simulink model "winder"  (R2025a)
settings: Solver=ode15s  StartTime=0.0  StopTime=Time.sim_time  FixedStep=Time.step_size  MaxStep=1e-4  RelTol=1e-3
values from neighbouring files (symbols this model uses):
  theta_table = Cam.theta_full    [winder_init.m]
  z_table = Cam.z_full    [winder_init.m]
undefined symbols (not defined in the file or in its folder): Cam, Core, Dancer, DC, Speed, Spool, Stepp, Tension, Wire
libraries: slpidlib x1
settings Model: Creator=psyco  LastModifiedBy=psyco

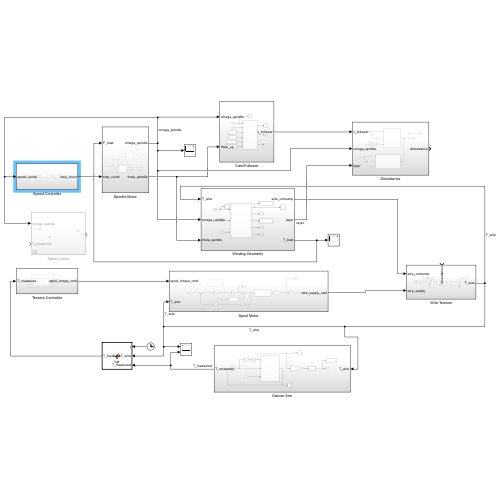
[thumbnail: Simulink's stored preview of the top-level diagram]
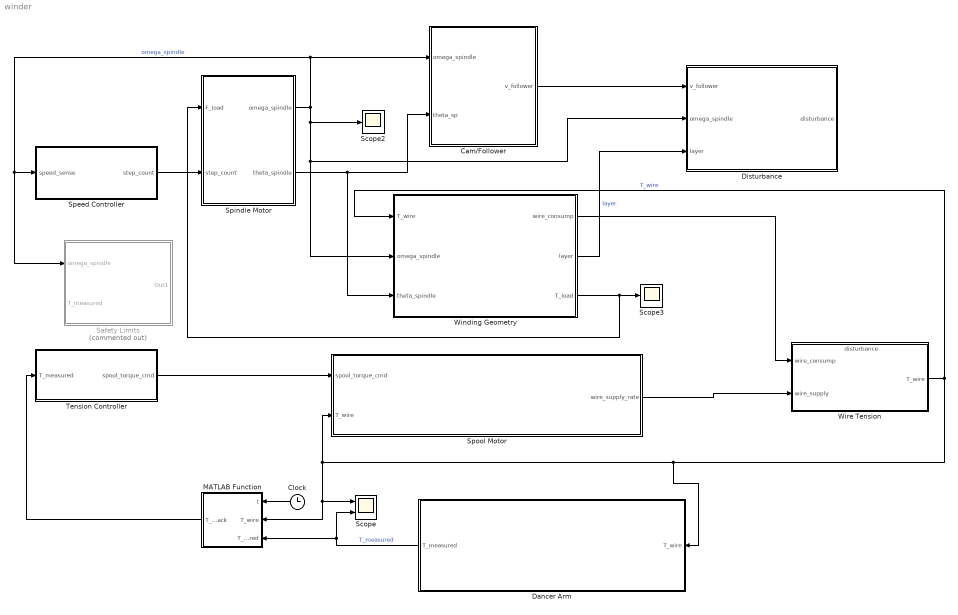
== system winder ==
  Cam/Follower : Subsystem
  Clock : Clock
  Dancer Arm : Subsystem
  Disturbance : Subsystem
  MATLAB Function : MATLAB Function  TreatAsAtomicUnit=on
  Safety Limits : Subsystem  Commented=on
  Scope : Scope  NumInputPorts=2
      settings: ActiveDisplayYMinimum=-0.018749999999999996  ActiveDisplayYMaximum=0.16874999999999998  DataLoggingVariableName=ScopeData4
  Scope2 : Scope
      settings: ActiveDisplayYMinimum=-0.006698983541536736  ActiveDisplayYMaximum=0.023139876765946442  DataLoggingVariableName=ScopeData3
  Scope3 : Scope
      settings: ActiveDisplayYMinimum=-1  ActiveDisplayYMaximum=1  DataLoggingVariableName=ScopeData8
  Speed Controller : Subsystem
  Spindle Motor : Subsystem
  Spool Motor : Subsystem
  Tension Controller : Subsystem
  Winding Geometry : Subsystem
  Wire Tension : Subsystem
      settings: PortSchema="{\"entries\":[{\"content\":{\"sides\":[{\"content\":{\"connectorIds\":[\"In1\",\"In2\"]},\"type\":\"ConnectorPlacement.EquallySpacedRectSide\",\"uuid\":\"81433370-ad2a-4528-8ca7-1fac031308da\"},{\"content\":{\"connectorIds\":[\"Out1\"],\"side\":\"RIGHT\"},\"type\":\"ConnectorPlacement.EquallySpacedRectSide\",\"uuid\":\"ed581ebd-7c4e-4c58-814b-bbfedd09dc09\"},{\"content\":{\"connectorIds\":[\"In3\"],\"side\":\"TOP\"},\"type\":\"ConnectorPlacement.EquallySpacedRectSide\",\"uuid\":\"8c939613-3eb5-48b9-810b-57417fa35655\"}]},\"type\":\"ConnectorPlacement.EquallySpacedConnector\",\"uuid\":\"39f3da8a-32c7-46ef-9441-56f9d7881147\"}],\"packageUris\":[\"http://schema.mathworks.com/mf0/Connector/R2020b\"],\"version\":\"1.0\"}"
  wires:
  Spindle Motor/2(theta_spindle) -> Cam/Follower/2(theta_sp), Winding Geometry/3(theta_spindle)
  Spindle Motor/1(omega_spindle) -> Winding Geometry/2(omega_spindle), Disturbance/2(omega_spindle), Scope2/1, Safety Limits/1(omega_spindle), Speed Controller/1(speed_sense), Cam/Follower/1(omega_spindle)  "omega_spindle"
  Winding Geometry/1(wire_consump) -> Wire Tension/1(wire_consump)
  Winding Geometry/2(layer) -> Disturbance/3(layer)  "layer"
  Winding Geometry/3(T_load) -> Spindle Motor/1(F_load), Scope3/1
  Cam/Follower/1(v_follower) -> Disturbance/1(v_follower)
  Speed Controller/1(step_count) -> Spindle Motor/2(step_count)
  Tension Controller/1(spool_torque_cmd) -> Spool Motor/1(spool_torque_cmd)
  Wire Tension/1(T_wire) -> Dancer Arm/1(T_wire), Scope/1, MATLAB Function/2(T_wire), Spool Motor/2(T_wire), Winding Geometry/1(T_wire)  "T_wire"
  Spool Motor/1(wire_supply_rate) -> Wire Tension/2(wire_supply)
  Dancer Arm/1(T_measured) -> MATLAB Function/3(T_measured), Scope/2  "T_measured"
  Clock/1 -> MATLAB Function/1(t)
  MATLAB Function/1(T_feedback) -> Tension Controller/1(T_measured)

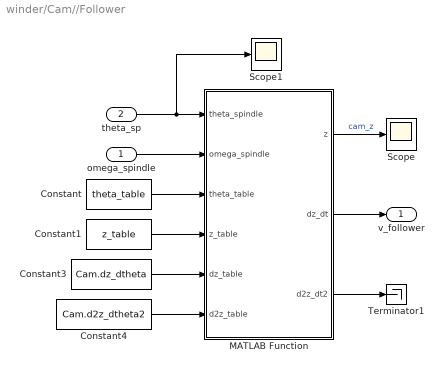
== system winder/Cam//Follower ==
  omega_spindle : Inport
  theta_sp : Inport  Port=2
  Constant : Constant  Value=theta_table
  Constant1 : Constant  Value=z_table
  Constant3 : Constant  Value=Cam.dz_dtheta
  Constant4 : Constant  Value=Cam.d2z_dtheta2
  MATLAB Function : MATLAB Function  TreatAsAtomicUnit=on
  Scope : Scope
      settings: ActiveDisplayYMinimum=-0.0087984481020212668  ActiveDisplayYMaximum=0.079186032918191415  DataLoggingVariableName=ScopeData6
  Scope1 : Scope
      settings: ActiveDisplayYMinimum=-1  ActiveDisplayYMaximum=1  DataLoggingVariableName=ScopeData7
  Terminator1 : Terminator
  v_follower : Outport
  wires:
  MATLAB Function/1(z) -> Scope/1  "cam_z"
  MATLAB Function/2(dz_dt) -> v_follower/1
  theta_sp/1 -> Scope1/1, MATLAB Function/1(theta_spindle)
  omega_spindle/1 -> MATLAB Function/2(omega_spindle)
  MATLAB Function/3(d2z_dt2) -> Terminator1/1
  Constant/1 -> MATLAB Function/3(theta_table)
  Constant1/1 -> MATLAB Function/4(z_table)
  Constant3/1 -> MATLAB Function/5(dz_table)
  Constant4/1 -> MATLAB Function/6(d2z_table)

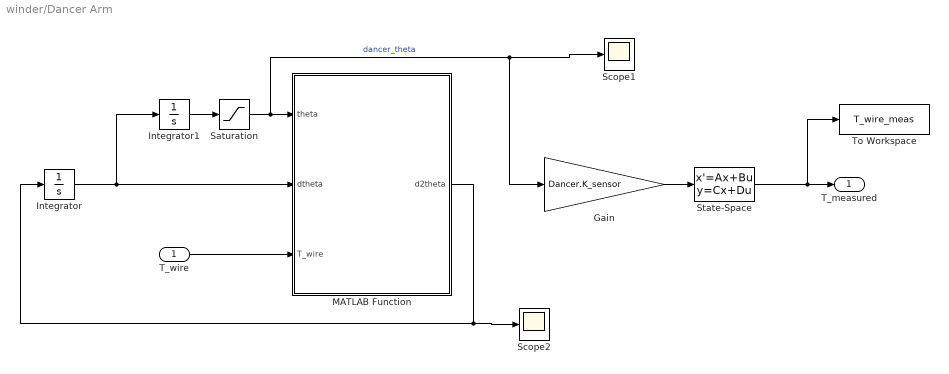
== system winder/Dancer Arm ==
  T_wire : Inport
  Gain : Gain  Gain=Dancer.K_sensor
  Integrator : Integrator  InitialCondition=0.0
  Integrator1 : Integrator  InitialCondition=Dancer.theta_IC
  MATLAB Function : MATLAB Function  TreatAsAtomicUnit=on
  Saturation : Saturate  UpperLimit=Dancer.theta_max  LowerLimit=Dancer.theta_min
  Scope1 : Scope
      settings: ActiveDisplayYMinimum=0.0653317811864291  ActiveDisplayYMaximum=0.14200863694398536  DataLoggingVariableName=ScopeData16
  Scope2 : Scope
      settings: ActiveDisplayYMinimum=-1  ActiveDisplayYMaximum=1  DataLoggingVariableName=ScopeData17
  State-Space : StateSpace  A=Dancer.A  B=Dancer.B  C=Dancer.C  D=Dancer.D  InitialCondition=Wire.T_pre/Dancer.C
  To Workspace : ToWorkspace  VariableName=T_wire_meas  SaveFormat=Timeseries  SampleTime=-1
  T_measured : Outport
  wires:
  T_wire/1 -> MATLAB Function/3(T_wire)
  MATLAB Function/1(d2theta) -> Scope2/1, Integrator/1
  Integrator/1 -> MATLAB Function/2(dtheta), Integrator1/1
  Integrator1/1 -> Saturation/1
  Saturation/1 -> Gain/1, Scope1/1, MATLAB Function/1(theta)  "dancer_theta"
  Gain/1 -> State-Space/1
  State-Space/1 -> To Workspace/1, T_measured/1

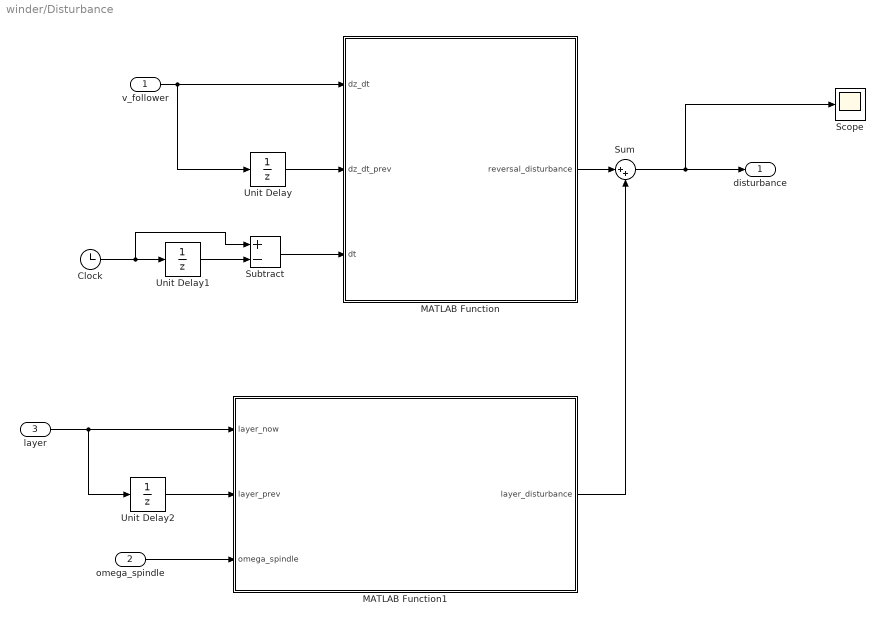
== system winder/Disturbance ==
  v_follower : Inport
  omega_spindle : Inport  Port=2
  layer : Inport  Port=3
  Clock : Clock
  MATLAB Function : MATLAB Function  TreatAsAtomicUnit=on
  MATLAB Function1 : MATLAB Function  TreatAsAtomicUnit=on
  Scope : Scope
      settings: ActiveDisplayYMinimum=-1  ActiveDisplayYMaximum=1  DataLoggingVariableName=ScopeData15
  Subtract : Sum  Inputs=+-
  Sum : Sum  Inputs=|++
  Unit Delay : UnitDelay  SampleTime=-1  HasFrameUpgradeWarning=on
  Unit Delay1 : UnitDelay  SampleTime=-1  HasFrameUpgradeWarning=on
  Unit Delay2 : UnitDelay  SampleTime=-1  HasFrameUpgradeWarning=on
  disturbance : Outport
  wires:
  v_follower/1 -> Unit Delay/1, MATLAB Function/1(dz_dt)
  Unit Delay/1 -> MATLAB Function/2(dz_dt_prev)
  Clock/1 -> Subtract/1, Unit Delay1/1
  Unit Delay1/1 -> Subtract/2
  Subtract/1 -> MATLAB Function/3(dt)
  layer/1 -> Unit Delay2/1, MATLAB Function1/1(layer_now)
  Unit Delay2/1 -> MATLAB Function1/2(layer_prev)
  omega_spindle/1 -> MATLAB Function1/3(omega_spindle)
  Sum/1 -> Scope/1, disturbance/1
  MATLAB Function/1(reversal_disturbance) -> Sum/1
  MATLAB Function1/1(layer_disturbance) -> Sum/2

== system winder/Safety Limits ==
  omega_spindle : Inport
  T_measured : Inport  Port=2
  Out1 : Outport

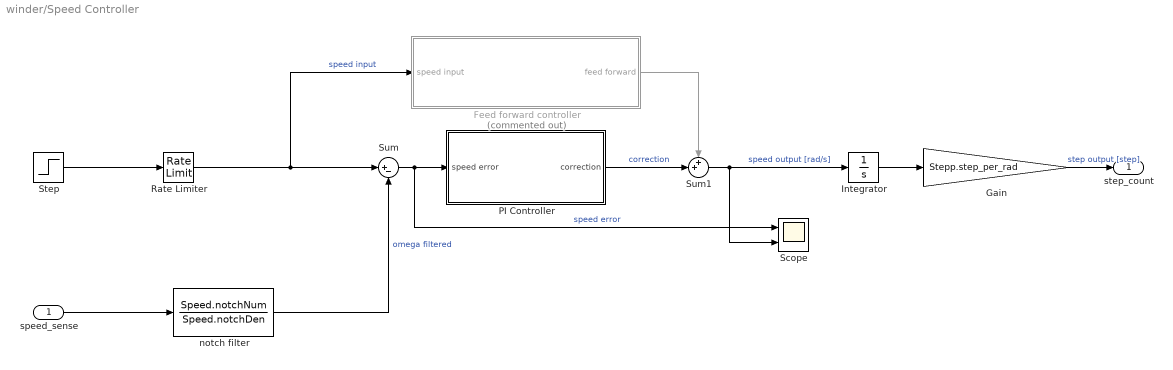
== system winder/Speed Controller ==
  speed_sense : Inport
  Feed forward controller : Subsystem  Commented=on
  Gain : Gain  Gain=Stepp.step_per_rad
  Integrator : Integrator  InitialCondition=0.0001  LimitOutput=on  UpperSaturationLimit=Stepp.omega_max  LowerSaturationLimit=-Stepp.omega_max
  PI Controller : Subsystem
  Rate Limiter : RateLimiter  RisingSlewLimit=Stepp.max_accel  FallingSlewLimit=-Stepp.max_accel  SampleTimeMode=inherited
  Scope : Scope  NumInputPorts=2
      settings: ActiveDisplayYMinimum=-0.012535486646997938  ActiveDisplayYMaximum=0.019935448467202885  DataLoggingVariableName=ScopeData10
  Step : Step  Time=0.1  After=Stepp.omega_target  SampleTime=0
  Sum : Sum  Inputs=|+-
  Sum1 : Sum  Inputs=++|
  notch filter : TransferFcn  Numerator=Speed.notchNum  Denominator=Speed.notchDen
  step_count : Outport
  wires:
  Step/1 -> Rate Limiter/1
  speed_sense/1 -> notch filter/1
  Rate Limiter/1 -> Feed forward controller/1(speed input), Sum/1  "speed input"
  Sum/1 -> Scope/1, PI Controller/1(speed error)  "speed error"
  Sum1/1 -> Integrator/1, Scope/2  "speed output [rad/s]"
  PI Controller/1(correction) -> Sum1/2  "correction"
  Gain/1 -> step_count/1  "step output [step]"
  notch filter/1 -> Sum/2  "omega filtered"
  Feed forward controller/1(feed forward) -> Sum1/1
  Integrator/1 -> Gain/1

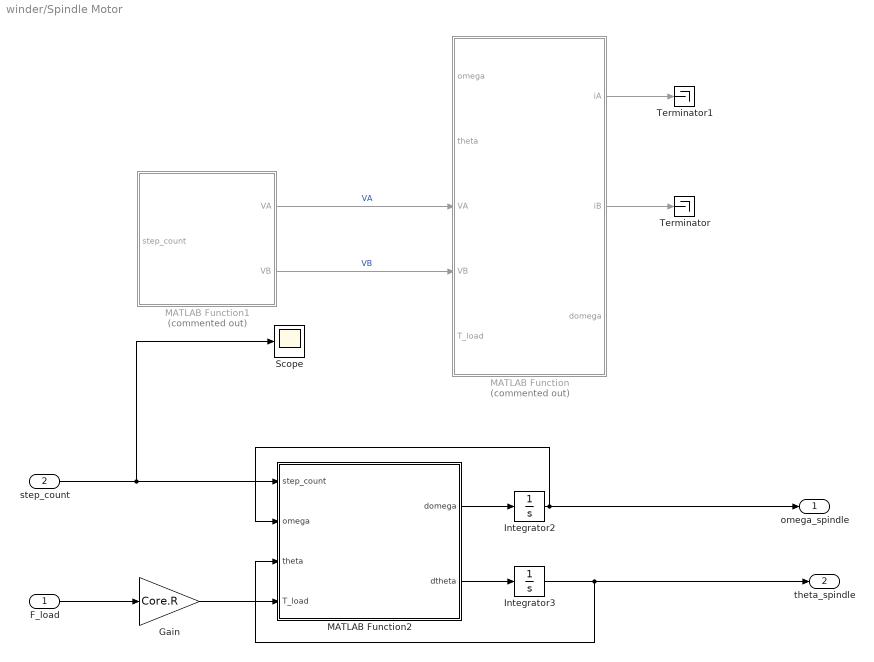
== system winder/Spindle Motor ==
  F_load : Inport
  step_count : Inport  Port=2
  Gain : Gain  Gain=Core.R
  Integrator2 : Integrator
  Integrator3 : Integrator
  MATLAB Function : MATLAB Function  Commented=on  TreatAsAtomicUnit=on
  MATLAB Function1 : MATLAB Function  Commented=on  TreatAsAtomicUnit=on
  MATLAB Function2 : MATLAB Function  TreatAsAtomicUnit=on
  Scope : Scope
      settings: ActiveDisplayYMinimum=-1  ActiveDisplayYMaximum=1  DataLoggingVariableName=ScopeData12
  Terminator : Terminator
  Terminator1 : Terminator
  omega_spindle : Outport
  theta_spindle : Outport  Port=2
  wires:
  step_count/1 -> Scope/1, MATLAB Function2/1(step_count)
  F_load/1 -> Gain/1
  Integrator2/1 -> MATLAB Function2/2(omega), omega_spindle/1
  Integrator3/1 -> theta_spindle/1, MATLAB Function2/3(theta)
  MATLAB Function1/1(VA) -> MATLAB Function/3(VA)  "VA"
  MATLAB Function1/2(VB) -> MATLAB Function/4(VB)  "VB"
  MATLAB Function/2(iB) -> Terminator/1
  MATLAB Function/1(iA) -> Terminator1/1
  MATLAB Function2/1(domega) -> Integrator2/1
  MATLAB Function2/2(dtheta) -> Integrator3/1
  Gain/1 -> MATLAB Function2/4(T_load)

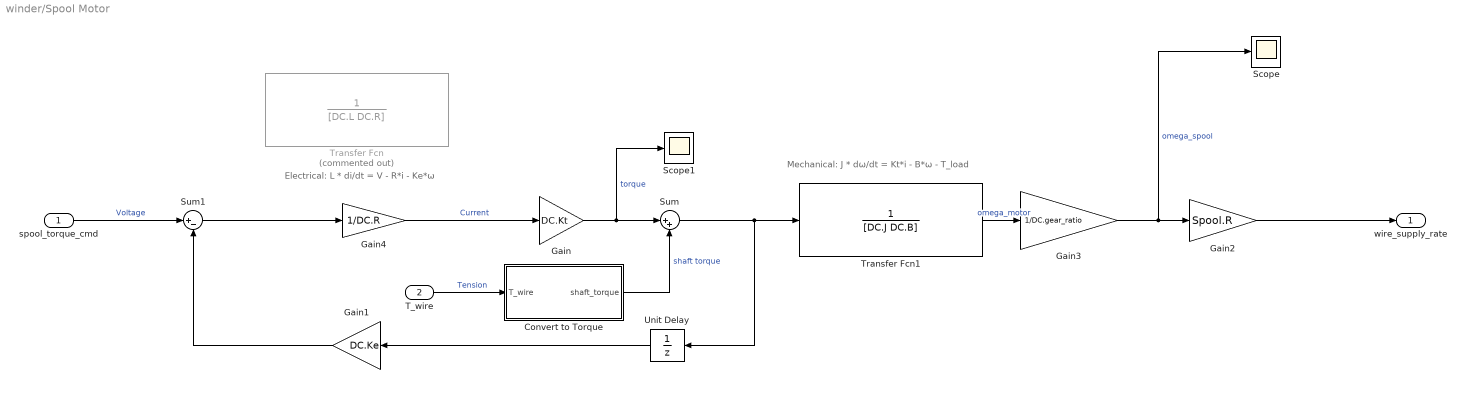
== system winder/Spool Motor ==
  note: Mechanical: J * dω/dt = Kt*i - B*ω - T_load
  note: Electrical: L * di/dt = V - R*i - Ke*ω
  spool_torque_cmd : Inport
  T_wire : Inport  Port=2
  Convert to Torque : Subsystem
  Gain : Gain  Gain=DC.Kt
  Gain1 : Gain  Gain=DC.Ke
  Gain2 : Gain  Gain=Spool.R
  Gain3 : Gain  Gain=1/DC.gear_ratio
  Gain4 : Gain  Gain=1/DC.R
  Scope : Scope
      settings: ActiveDisplayYMinimum=-0.32096795666612027  ActiveDisplayYMaximum=0.063976217926597662
  Scope1 : Scope
      settings: ActiveDisplayYMinimum=-1  ActiveDisplayYMaximum=1  DataLoggingVariableName=ScopeData13
  Sum : Sum  Inputs=|++
  Sum1 : Sum  Inputs=|+-
  Transfer Fcn : TransferFcn  Commented=on  Denominator=[DC.L DC.R]
  Transfer Fcn1 : TransferFcn  Denominator=[DC.J DC.B]
  Unit Delay : UnitDelay  SampleTime=-1  HasFrameUpgradeWarning=on
  wire_supply_rate : Outport
  wires:
  spool_torque_cmd/1 -> Sum1/1  "Voltage"
  Gain4/1 -> Gain/1  "Current"
  Gain/1 -> Scope1/1, Sum/1  "torque"
  Sum/1 -> Unit Delay/1, Transfer Fcn1/1
  Sum1/1 -> Gain4/1
  Gain1/1 -> Sum1/2
  Gain3/1 -> Scope/1, Gain2/1  "omega_spool"
  Transfer Fcn1/1 -> Gain3/1  "omega_motor"
  T_wire/1 -> Convert to Torque/1(T_wire)  "Tension"
  Convert to Torque/1(shaft_torque) -> Sum/2  "shaft torque"
  Unit Delay/1 -> Gain1/1
  Gain2/1 -> wire_supply_rate/1

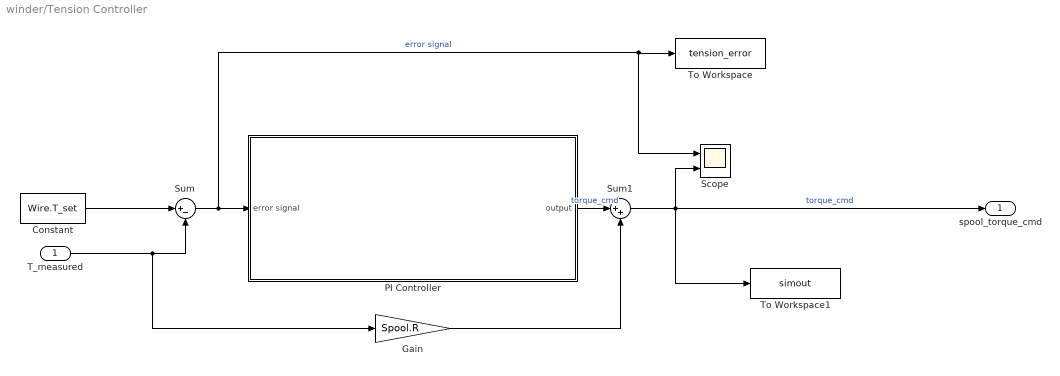
== system winder/Tension Controller ==
  T_measured : Inport
  Constant : Constant  Value=Wire.T_set
  Gain : Gain  Gain=Spool.R
  PI Controller : Subsystem
  Scope : Scope  NumInputPorts=2
      settings: ActiveDisplayYMinimum=-0.28301132150109948  ActiveDisplayYMaximum=0.10780803609590808
  Sum : Sum  Inputs=|+-
  Sum1 : Sum  Inputs=|++
  To Workspace : ToWorkspace  VariableName=tension_error  SaveFormat=Timeseries  SampleTime=-1
  To Workspace1 : ToWorkspace  VariableName=simout  SaveFormat=Timeseries  SampleTime=-1
  spool_torque_cmd : Outport
  wires:
  Constant/1 -> Sum/1
  Sum/1 -> Scope/1, To Workspace/1, PI Controller/1(error signal)  "error signal"
  T_measured/1 -> Gain/1, Sum/2
  Sum1/1 -> spool_torque_cmd/1, To Workspace1/1, Scope/2  "torque_cmd"
  PI Controller/1(output) -> Sum1/1  "torque_cmd"
  Gain/1 -> Sum1/2

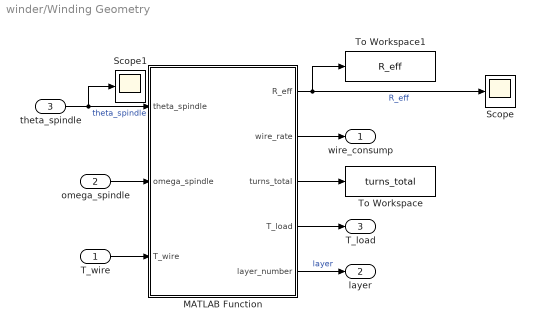
== system winder/Winding Geometry ==
  T_wire : Inport
  omega_spindle : Inport  Port=2
  theta_spindle : Inport  Port=3
  MATLAB Function : MATLAB Function  TreatAsAtomicUnit=on
  Scope : Scope
      settings: ActiveDisplayYMinimum=0.0042724999999999994  ActiveDisplayYMaximum=0.0072475  DataLoggingVariableName=ScopeData5
  Scope1 : Scope
      settings: ActiveDisplayYMinimum=-0.00057455487689339743  ActiveDisplayYMaximum=0.0051554766735195058  DataLoggingVariableName=ScopeData2
  To Workspace : ToWorkspace  VariableName=turns_total  SaveFormat=Timeseries  SampleTime=-1
  To Workspace1 : ToWorkspace  VariableName=R_eff  SaveFormat=Timeseries  SampleTime=-1
  wire_consump : Outport
  layer : Outport  Port=2
  T_load : Outport  Port=3
  wires:
  MATLAB Function/1(R_eff) -> To Workspace1/1, Scope/1  "R_eff"
  MATLAB Function/2(wire_rate) -> wire_consump/1
  MATLAB Function/5(layer_number) -> layer/1  "layer"
  theta_spindle/1 -> Scope1/1, MATLAB Function/1(theta_spindle)  "theta_spindle"
  omega_spindle/1 -> MATLAB Function/2(omega_spindle)
  T_wire/1 -> MATLAB Function/3(T_wire)
  MATLAB Function/4(T_load) -> T_load/1
  MATLAB Function/3(turns_total) -> To Workspace/1

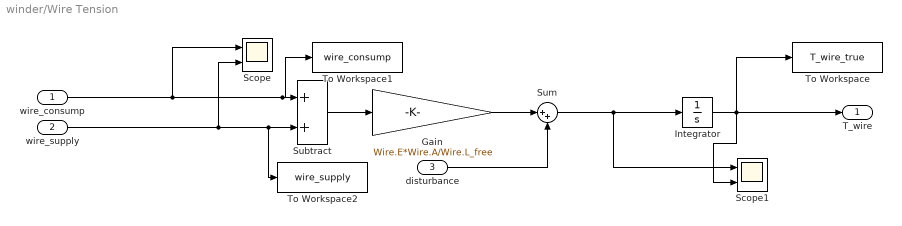
== system winder/Wire Tension ==
  wire_consump : Inport
  wire_supply : Inport  Port=2
  disturbance : Inport  Port=3
  Gain : Gain  Gain=Wire.E*Wire.A/Wire.L_free
  Integrator : Integrator  InitialCondition=Wire.T_pre  LimitOutput=on  UpperSaturationLimit=Wire.T_max  LowerSaturationLimit=0
  Scope : Scope  NumInputPorts=2
      settings: ActiveDisplayYMinimum=-0.0013474271478965518  ActiveDisplayYMaximum=0.0014312796853598328  DataLoggingVariableName=ScopeData9
  Scope1 : Scope  NumInputPorts=2
      settings: ActiveDisplayYMinimum=-1  ActiveDisplayYMaximum=1  DataLoggingVariableName=ScopeData14
  Subtract : Sum
  Sum : Sum  Inputs=|++
  To Workspace : ToWorkspace  VariableName=T_wire_true  SaveFormat=Timeseries  SampleTime=-1
  To Workspace1 : ToWorkspace  VariableName=wire_consump  SaveFormat=Timeseries  SampleTime=-1
  To Workspace2 : ToWorkspace  VariableName=wire_supply  SaveFormat=Timeseries  SampleTime=-1
  T_wire : Outport
  wires:
  wire_consump/1 -> Scope/1, To Workspace1/1, Subtract/1
  wire_supply/1 -> Scope/2, To Workspace2/1, Subtract/2
  Gain/1 -> Sum/1
  Integrator/1 -> To Workspace/1, Scope1/2, T_wire/1
  Sum/1 -> Scope1/1, Integrator/1
  disturbance/1 -> Sum/2
  Subtract/1 -> Gain/1

== system winder/Speed Controller/Feed forward controller ==
  speed input : Inport
  Gain : Gain  Gain=Stepp.step_per_rev
  Gain1 : Gain  Gain=1/(2*pi)
  feed forward : Outport
  wires:
  Gain/1 -> Gain1/1
  speed input/1 -> Gain/1
  Gain1/1 -> feed forward/1  "feed forward"

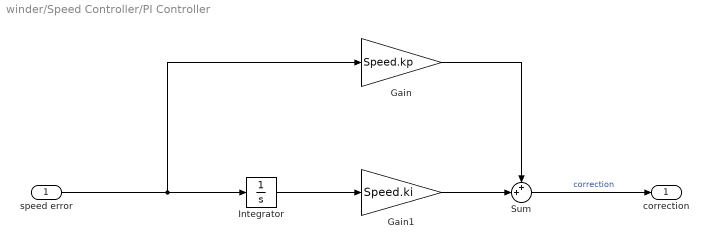
== system winder/Speed Controller/PI Controller ==
  speed error : Inport
  Gain : Gain  Gain=Speed.kp
  Gain1 : Gain  Gain=Speed.ki
  Integrator : Integrator  WrapState=on  WrappedStateUpperValue=Speed.AW_limit  WrappedStateLowerValue=-Speed.AW_limit
  Sum : Sum  Inputs=++|
  correction : Outport
  wires:
  speed error/1 -> Integrator/1, Gain/1
  Sum/1 -> correction/1  "correction"
  Integrator/1 -> Gain1/1
  Gain1/1 -> Sum/2
  Gain/1 -> Sum/1

== system winder/Spool Motor/Convert to Torque ==
  T_wire : Inport
  Gain4 : Gain  Gain=Spool.R/DC.gear_ratio/DC.eta_gearbox
  shaft_torque : Outport
  wires:
  Gain4/1 -> shaft_torque/1
  T_wire/1 -> Gain4/1

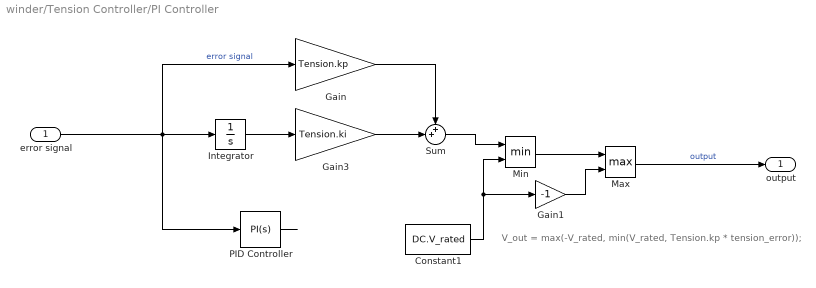
== system winder/Tension Controller/PI Controller ==
  note: V_out = max(-V_rated, min(V_rated, Tension.kp * tension_error));
  error signal : Inport
  Constant1 : Constant  Value=DC.V_rated
  Gain : Gain  Gain=Tension.kp
  Gain1 : Gain  Gain=-1
  Gain3 : Gain  Gain=Tension.ki
  Integrator : Integrator
  Max : MinMax  Function=max  Inputs=2
  Min : MinMax  Inputs=2
  PID Controller : slpidlib/PID Controller  Controller=PI  Form=Parallel  TimeDomain=Continuous-time  UseExternalTs=off  SampleTime=-1  IntegratorMethod=Forward Euler  FilterMethod=Forward Euler  ControllerParametersSource=internal  P=Tension.kp  I=Tension.ki  UseKiTs=off  D=0  UseExternalDerivativeSource=off  N=100  UseFilter=on  TunerSelectOption=Transfer Function Based (PID Tuner App)  InitialConditionSource=internal  InitialConditionForIntegrator=0  InitialConditionForFilter=0  DifferentiatorICPrevScaledInput=0  ExternalReset=none  TrackingMode=off  Kt=1  LimitOutput=off  SatLimitsSource=internal  UpperSaturationLimit=inf  LowerSaturationLimit=-inf  LinearizeAsGain=on  AntiWindupMode=none  Kb=1  LimitIntegrator=off  UpperIntegratorSaturationLimit=inf  LowerIntegratorSaturationLimit=-inf  POutMin=[]  POutMax=[]  IOutMin=[]  IOutMax=[]  DOutMin=[]  DOutMax=[]  NOutMin=[]  NOutMax=[]  SumOutMin=[]  SumOutMax=[]  SaturationOutMin=[]  SaturationOutMax=[]  PParamMin=[]  PParamMax=[]  IParamMin=[]  IParamMax=[]  DParamMin=[]  DParamMax=[]  NParamMin=[]  NParamMax=[]  KbParamMin=[]  KbParamMax=[]  KtParamMin=[]  KtParamMax=[]  KbOutMin=[]  KbOutMax=[]  KtOutMin=[]  KtOutMax=[]  IntegratorOutMin=[]  IntegratorOutMax=[]  FilterOutMin=[]  FilterOutMax=[]  SumI1OutMin=[]  SumI1OutMax=[]  SumI2OutMin=[]  SumI2OutMax=[]  SumI3OutMin=[]  SumI3OutMax=[]  SumI4OutMin=[]  SumI4OutMax=[]  SumDOutMin=[]  SumDOutMax=[]  DifferentiatorOutMin=[]  DifferentiatorOutMax=[]  FilterDiffOutCoefMin=[]  FilterDiffOutCoefMax=[]  ReciprocalOutMin=[]  ReciprocalOutMax=[]  SumDenOutMin=[]  SumDenOutMax=[]  SumNumOutMin=[]  SumNumOutMax=[]  DivideOutMin=[]  DivideOutMax=[]  UdiffTsProdOutMin=[]  UdiffTsProdOutMax=[]  NTsProdOutMin=[]  NTsProdOutMax=[]  UintegralTsProdOutMin=[]  UintegralTsProdOutMax=[]  UngainTsProdOutMin=[]  UngainTsProdOutMax=[]  ClampingZeroOutDataTypeStr=Inherit: Inherit via back propagation  ClampingZeroOutMin=[]  ClampingZeroOutMax=[]  FilterDenConstantOutDataTypeStr=Inherit: Inherit via back propagation  FilterDenConstantOutMin=[]  FilterDenConstantOutMax=[]  PCopyOutDataTypeStr=Inherit: Inherit via back propagation  PCopyOutMin=[]  PCopyOutMax=[]  NCopyOutDataTypeStr=Inherit: Inherit via back propagation  NCopyOutMin=[]  NCopyOutMax=[]  IntegratorContinuousStateAttributes=''  IntegratorStateMustResolveToSignalObject=off  IntegratorRTWStateStorageClass=Auto  FilterContinuousStateAttributes=''  FilterStateMustResolveToSignalObject=off  FilterRTWStateStorageClass=Auto  ParallelPVariant=InternalParameters  IdealPVariant=Disabled  IVariant=InternalParameters  DVariant=Disabled  IntegratorVariant=Continuous  SatVariant=Disabled  AWVariant=Passthrough  PCopyVariant=Disabled  TRVariant=Disabled  FdbkBlocksVariant=Forward  IdealPFdbkVariant=Disabled  SatFdbkVariant=Disabled  DerivativeFilterVariant=Disabled  NVariant=Disabled  NCopyVariant=Disabled_SignalSpec  FilterICVariant=Disabled  IntegratorICVariant=InternalICs  ExternalResetVariant=Disabled  TRSumVariant=Passthrough  SumFdbkVariant=Disabled  SumVariant=Sum_PI  TsampFilterVariant=InternalTs  TsampNgainVariant=Passthrough  TsampIntegralVariant=Disabled_SignalSpec  ExternalSaturationOutDataTypeStr=Inherit: Same as second input  DerivativeSourceVariant=Disabled  PreIntVariant=InternalPreInt
  Sum : Sum  Inputs=++|
  output : Outport
  wires:
  Min/1 -> Max/1
  Gain1/1 -> Max/2
  Gain/1 -> Sum/1
  Max/1 -> output/1  "output"
  Constant1/1 -> Min/2, Gain1/1
  error signal/1 -> PID Controller/1, Integrator/1, Gain/1  "error signal"
  PID Controller/1 -> ?
  Integrator/1 -> Gain3/1
  Gain3/1 -> Sum/2
  Sum/1 -> Min/1

== matlab function winder/Spindle Motor/MATLAB Function2 ==
  data: step_count input; domega output; omega input; theta input; T_load input; dtheta output; Stepp parameter
function [domega, dtheta] = stepper_simplified(step_count, omega, theta, T_load, Stepp)
    % Parameters
    microstep_divisor = Stepp.microstep_divisor;
    step_angle = 2*pi / (200 * microstep_divisor);  % rad per microstep
    
    % 1. Calculate commanded position
    theta_commanded = step_count * step_angle;
    
    % 2. Position error (wrap to -pi to pi)
    theta_error = theta_commanded - theta;
    theta_error = mod(theta_error + pi, 2*pi) - pi;
    
    % 3. Electromagnetic Torque (Linear Spring Approximation)
    % A real stepper is T_hold * sin(Nr * theta_error). 
    % For small errors, sin(x) ~ x. This linear version is much more 
    % stable for Simulink solvers at 0.005s step sizes.
    T_hold = Stepp.Kt * Stepp.I_rated;       % Approx holding torque
    K_spring = T_hold * Stepp.Nr;            % Effective torsional stiffness (Nm/rad)
    
    T_electromagnetic = K_spring * theta_error;
    
    % Saturation (The motor can't produce more than holding torque)
    T_electromagnetic = max(min(T_electromagnetic, T_hold), -T_hold);
    
    % 4. Virtual Damping (Crucial for stability)
    % The physical B is tiny, but the numerical spring is stiff.
    % We calculate critical damping and use a fraction of it to prevent 
    % the 200Hz numerical chatter while keeping the system responsive.
    B_critical = 2 * sqrt(K_spring * Stepp.J);
    B_virtual = 0.5 * B_critical; % 30% of critical damping
    
    % Total damping = Physical + Virtual
    B_total = Stepp.B + B_virtual;
    
    % 5. Mechanical Dynamics
    % J*domega/dt = T_motor - T_load - B*omega
    domega = (T_electromagnetic - T_load - B_total * omega) / Stepp.J;
    dtheta = omega;
end

== matlab function winder/MATLAB Function ==
  data: t input; T_feedback output; T_wire input; T_measured input
function T_feedback = fcn(t,T_wire,T_measured)

a = t-1;
T_feedback = (1-a)*T_wire + a*T_measured;
end

== matlab function winder/Spindle Motor/MATLAB Function1 ==
  data: step_count input; VA output; VB output; Stepp parameter
function [VA, VB] = stepper_driver(step_count, Stepp)
    I_rated = Stepp.I_rated;
    R_phase = Stepp.R_phase;
    microstep_divisor = Stepp.microstep_divisor;
    
    theta_elec = step_count * (2*pi / (4 * microstep_divisor));
    
    % Calculate voltage required to drive I_rated through R_phase
    % V = I * R
    V_target = I_rated * R_phase; 
    
    % Sinusoidal microstepping
    VA = V_target * cos(theta_elec);
    VB = V_target * sin(theta_elec);
    
    % Clip to supply voltage (just in case)
    VA = max(min(VA, Stepp.V_supp), -Stepp.V_supp);
    VB = max(min(VB, Stepp.V_supp), -Stepp.V_supp);
end

== matlab function winder/Spindle Motor/MATLAB Function ==
  data: iA output; omega input; theta input; VA input; VB input; T_load input; iB output; domega output; Stepp parameter
function [iA, iB, domega] = stepper_derivatives(omega, theta, VA, VB, T_load, Stepp)
    Nr = Stepp.Nr;     % rotor teeth = 50
    R  = Stepp.R_phase;      % phase resistance, [Ohms]
    % L  = Stepp.L;      % phase inductance, [H]
    Ke = Stepp.Ke;     % back-EMF constant
    Kt = Stepp.Kt;     % torque constant
    J  = Stepp.J;      % rotor inertia, [kgm^2]
    B  = Stepp.B;      % damping

    % Electrical equations
    % diA = (VA - R*iA - Ke*omega*sin(Nr*theta)) / L;
    % diB = (VB - R*iB + Ke*omega*cos(Nr*theta)) / L;
    iA = (VA - Ke*omega*sin(Nr*theta)) / R;
    iB = (VB - Ke*omega*cos(Nr*theta)) / R;
    % Mechanical equation
    T_em = Kt * (iA*sin(Nr*theta) - iB*cos(Nr*theta));
    domega = (T_em - B*omega - T_load) / J;
end

== matlab function winder/Winding Geometry/MATLAB Function ==
  data: theta_spindle input; R_eff output; omega_spindle input; T_wire input; wire_rate output; turns_total output; T_load output; layer_number output; Wire parameter; Core parameter; Cam parameter
function [R_eff, wire_rate, turns_total, T_load, layer_number] = ...
         winding_geometry(theta_spindle, omega_spindle, T_wire, Wire, Core, Cam)

    % Unpack parameters
    R_core          = Core.R;
    wire_d          = Wire.diam;
    gear_reduction = Cam.gear_ratio;

    % Total turns from spindle angle
    turns_total = theta_spindle / (2*pi);
    cam_cycles = theta_spindle/(12*pi*gear_reduction); % Beta*gear_reduction

    % Current layer (zero-indexed)
    layer_number = max(0,floor(cam_cycles));

    % Current effective winding radius
    R_eff = R_core + (layer_number + 0.5) * wire_d;
    % +0.5 puts R_eff at the midpoint of the current layer

    % Wire consumption rate (m/s)
    % Arc length per radian * angular velocity
    wire_rate = R_eff * omega_spindle;

    % Torque load on spindle from wire tension
    T_load = T_wire * R_eff;
end

== matlab function winder/Cam//Follower/MATLAB Function ==
  data: theta_spindle input; z output; omega_spindle input; theta_table input; z_table input; dz_table input; d2z_table input; dz_dt output; d2z_dt2 output; Cam parameter
function [z, dz_dt, d2z_dt2] = cam_follower_csv(theta_spindle, omega_spindle,...
                theta_table, z_table, dz_table, d2z_table,Cam)
    
    gear_ratio = Cam.gear_ratio;
    
    % if isempty(cam_interp)
    %     % Load the two groove CSVs
    %     rise_data   = readmatrix('cam_groove1.csv');    % [x, y, z] columns
    %     return_data = readmatrix('cam_groove2.csv');
    %     % Extract axial position (z column) and compute cam angle from x,y
    %     % Since x = R*cos(theta), y = R*sin(theta):        
    %     theta_rise   = atan2(rise_data(:,2), rise_data(:,1)); % [rad]
    %     theta_return = atan2(return_data(:,2), return_data(:,1)); % [rad]
    % 
    %     z_rise_raw   = rise_data(:,3)*1e-2;    % convert cm to [m]
    %     z_return_raw = return_data(:,3)*1e-2;
    % 
    %     % Remove offset
    %     z_rise = z_rise_raw - z_rise_raw(1);
    %     z_return = z_return_raw - z_return_raw(1);
    % 
    %     % Flip return
    %     z_return = max(z_rise) + z_return;
    % 
    %     % Unwrap angles to make them monotonically increasing
    %     theta_rise   = unwrap(theta_rise);
    %     theta_return = unwrap(theta_return);
    % 
    %     % Shift return angles to start where rise ends (at 2*pi)
    %     theta_return = theta_return - theta_return(1) + ...
    %                         theta_rise(end);
    % 
    %     % Concatenate into one full cycle table (0 to 4*pi)
    %     theta_full = [theta_rise; theta_return];
    %     z_full     = [z_rise; z_return];
    % 
    %     % Remove duplicate theta values
    %     [theta_full, unique_idx] = unique(theta_full, 'stable');
    %     z_full = z_full(unique_idx);
    % 
    %     % Verify monotonically increasing (griddedInterpolant requires this)
    %     if any(diff(theta_full) <= 0)
    %         % Sort to enforce monotonic order
    %         [theta_full, sort_idx] = sort(theta_full);
    %         z_full = z_full(sort_idx);
    %     end
    % 
    % 
    %     theta_table = theta_full;
    %     z_table = z_full;
    % end

    % Cam angle, normalized to one full cycle
    theta_cam   = theta_spindle / gear_ratio;
    theta_cycle = mod(theta_cam, 24*pi);
    omega_cam   = omega_spindle / gear_ratio;

    % Small perturbation for numerical derivatives
    % dtheta = 1e-4;

    % % Position
    % z = interp1(theta_table, z_table, theta_cycle, 'linear');
    % z_plus  = interp1(theta_table, z_table, theta_cycle + dtheta,  'linear');
    % z_minus = interp1(theta_table, z_table, theta_cycle - dtheta,  'linear');
    % z_plus2 = interp1(theta_table, z_table, theta_cycle + 2*dtheta,'linear');
    % z_minus2= interp1(theta_table, z_table, theta_cycle - 2*dtheta,'linear');


    z        = interp1(theta_table, z_table, theta_cycle, 'linear');
    dz_dth   = interp1(theta_table, dz_table, theta_cycle, 'linear');
    d2z_dth2 = interp1(theta_table, d2z_table, theta_cycle, 'linear');

    dz_dt    = dz_dth * omega_cam;
    d2z_dt2  = d2z_dth2 * omega_cam^2;

    % reversal = abs(dz_dth) < 1e-3;

    % Velocity — numerical derivative of profile w.r.t. cam angle,
    % scaled by cam angular velocity
    % dz_dtheta   = (z_plus - z_minus) / (2*dtheta);
    % dz_dt = dz_dtheta * omega_cam;
    % 
    % % Acceleration — second derivative
    % d2z_dtheta2 = (z_plus2 - 2*z + z_minus2) / dtheta^2;
    % d2z_dt2 = d2z_dtheta2 * omega_cam^2;
end

== matlab function winder/Disturbance/MATLAB Function ==
  data: dz_dt input; reversal_disturbance output; dz_dt_prev input; dt input; Wire parameter
function reversal_disturbance = cam_reversal_disturbance(dz_dt, dz_dt_prev, dt, Wire)
    % Detect zero crossing in traversal velocity
    sign_change = sign(dz_dt) ~= sign(dz_dt_prev);
    near_zero   = abs(dz_dt) < 0.001;   % 0.001 m/s
    
    reversal_event = sign_change & near_zero;
    
    % Tension disturbance magnitude
    % Wire has to change direction -- creates a brief tension spike
    % proportional to wire stiffness and traversal velocity change
    delta_v = abs(dz_dt - dz_dt_prev);
    
    if reversal_event
        % Impulse magnitude -- wire spring constant * velocity change
        reversal_disturbance = Wire.K * delta_v * dt;
    else
        reversal_disturbance = 0;
    end
end

== matlab function winder/Disturbance/MATLAB Function1 ==
  data: layer_now input; layer_disturbance output; layer_prev input; omega_spindle input; Wire parameter
function layer_disturbance = layer_transition_disturbance(layer_now, layer_prev, ...
                                                           omega_spindle, Wire)
    layer_changed = layer_now > layer_prev;
    
    if layer_changed
        % Step change in wire consumption rate
        delta_R         = Wire.diam;         % 0.140e-3 m
        delta_wire_rate = omega_spindle * delta_R;      % m/s

        % Tension disturbance from sudden rate increase
        % Tension drops briefly as spool catches up
        layer_disturbance = -Wire.K * delta_wire_rate * Wire.tau_spool;
        % tau_spool is your spool motor response time, ~0.05-0.1s
    else
        layer_disturbance = 0;
    end
end

== matlab function winder/Dancer Arm/MATLAB Function ==
  data: theta input; dtheta input; T_wire input; d2theta output; Dancer parameter
function d2theta = dancer_arm_ode(theta, dtheta, T_wire, Dancer)
    torque_from_tension = 2*T_wire * Dancer.L_arm * cos(theta);  % or appropriate geometry
    d2theta = (torque_from_tension - Dancer.K_spring*theta - Dancer.B_crit*dtheta)...
                / Dancer.J_arm;
end
